simulink model "Bai02"  (R2023b)
settings: Solver=VariableStepAuto  StartTime=0.0  StopTime=0.1  RelTol=1e-3
settings Model: Creator=Trung  LastModifiedBy=Trung

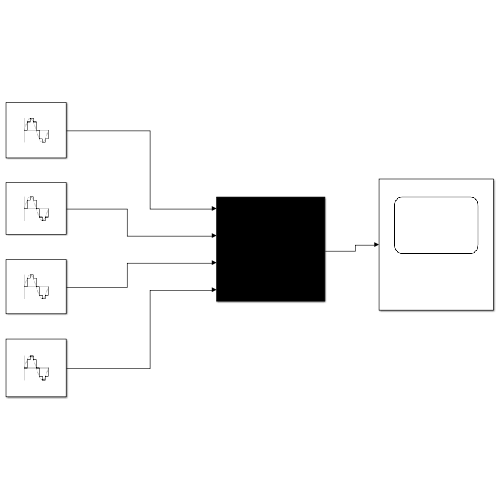
[thumbnail: Simulink's stored preview of the top-level diagram]
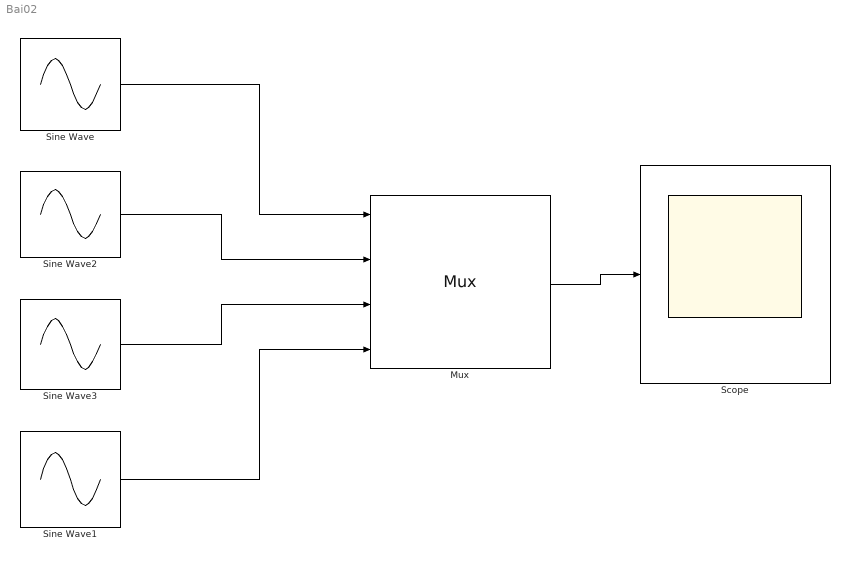
== system Bai02 ==
  Mux : Mux
  Scope : Scope
  Sine Wave : Sin  Frequency=2*pi*50  SampleTime=0.0001
  Sine Wave1 : Sin  Frequency=2*pi*50  Phase=1.5 * pi  SampleTime=0.0001
  Sine Wave2 : Sin  Frequency=2*pi*50  Phase=pi/2  SampleTime=0.0001
  Sine Wave3 : Sin  Frequency=2*pi*50  Phase=pi  SampleTime=0.0001
  wires:
  Sine Wave/1 -> Mux/1
  Sine Wave2/1 -> Mux/2
  Sine Wave3/1 -> Mux/3
  Sine Wave1/1 -> Mux/4
  Mux/1 -> Scope/1
